simulink model "Firmodel"  (R2023b)
settings: Solver=VariableStepAuto  StartTime=0.0  StopTime=10.0  RelTol=1e-3
values from neighbouring files (symbols this model uses):
  ts = 1/fs    (= 4e-05)    [FIR.m]    (also in FIRfiltSam.m)
settings Model: Creator=91798  LastModifiedBy=91798
settings DataIOCC: ReturnWorkspaceOutputs=off

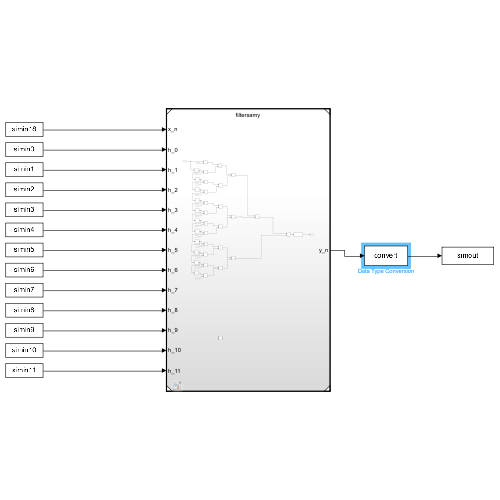
[thumbnail: Simulink's stored preview of the top-level diagram]
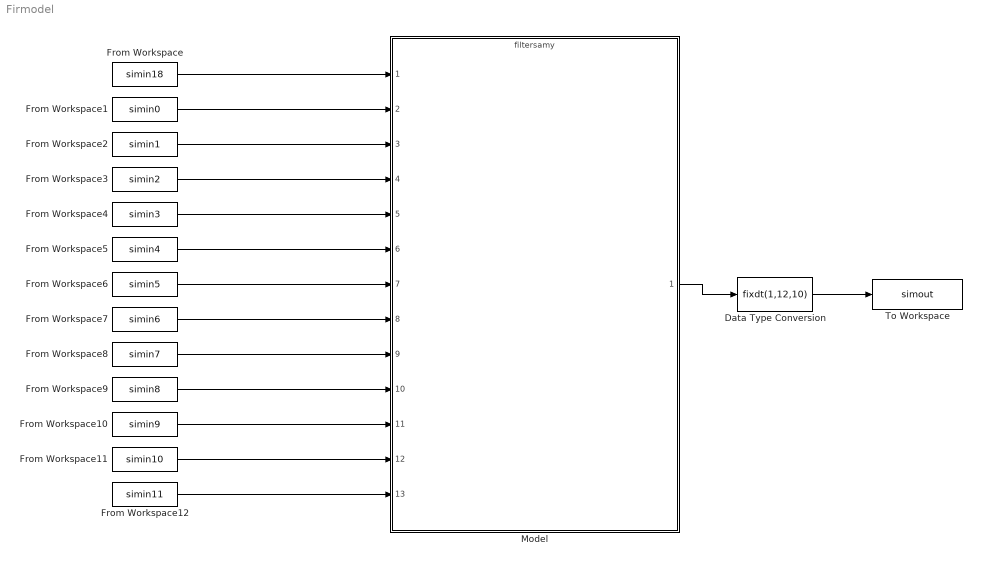
== system Firmodel ==
  Data Type Conversion : DataTypeConversion  OutDataTypeStr=fixdt(1,12,10)  SaturateOnIntegerOverflow=off  RndMeth=Floor
  From Workspace : FromWorkspace  VariableName=simin18  OutDataTypeStr=fixdt(1,8,6)  Interpolate=off  OutputAfterFinalValue=Setting to zero
  From Workspace1 : FromWorkspace  VariableName=simin0  OutDataTypeStr=fixdt(1,8,6)  Interpolate=off  OutputAfterFinalValue=Setting to zero
  From Workspace10 : FromWorkspace  VariableName=simin9  OutDataTypeStr=fixdt(1,8,6)  Interpolate=off  OutputAfterFinalValue=Setting to zero
  From Workspace11 : FromWorkspace  VariableName=simin10  OutDataTypeStr=fixdt(1,8,6)  SampleTime=ts  Interpolate=off  OutputAfterFinalValue=Setting to zero
  From Workspace12 : FromWorkspace  VariableName=simin11  OutDataTypeStr=fixdt(1,8,6)  Interpolate=off  OutputAfterFinalValue=Setting to zero
  From Workspace2 : FromWorkspace  VariableName=simin1  OutDataTypeStr=fixdt(1,8,6)  Interpolate=off  OutputAfterFinalValue=Setting to zero
  From Workspace3 : FromWorkspace  VariableName=simin2  OutDataTypeStr=fixdt(1,8,6)  Interpolate=off  OutputAfterFinalValue=Setting to zero
  From Workspace4 : FromWorkspace  VariableName=simin3  OutDataTypeStr=fixdt(1,8,6)  OutputAfterFinalValue=Setting to zero
  From Workspace5 : FromWorkspace  VariableName=simin4  OutDataTypeStr=fixdt(1,8,6)  Interpolate=off  OutputAfterFinalValue=Setting to zero
  From Workspace6 : FromWorkspace  VariableName=simin5  OutDataTypeStr=fixdt(1,8,6)  Interpolate=off  OutputAfterFinalValue=Setting to zero
  From Workspace7 : FromWorkspace  VariableName=simin6  OutDataTypeStr=fixdt(1,8,6)  Interpolate=off  OutputAfterFinalValue=Setting to zero
  From Workspace8 : FromWorkspace  VariableName=simin7  OutDataTypeStr=fixdt(1,8,6)  Interpolate=off  OutputAfterFinalValue=Setting to zero
  From Workspace9 : FromWorkspace  VariableName=simin8  OutDataTypeStr=fixdt(1,8,6)  Interpolate=off  OutputAfterFinalValue=Setting to zero
  Model : ModelReference  ModelNameDialog=filtersamy.slx  SimulationMode=Normal  ModelReferenceVersion=2.5
  To Workspace : ToWorkspace  VariableName=simout  SaveFormat=Timeseries  SampleTime=-1
  wires:
  From Workspace/1 -> Model/1
  From Workspace1/1 -> Model/2
  From Workspace2/1 -> Model/3
  From Workspace3/1 -> Model/4
  From Workspace4/1 -> Model/5
  From Workspace5/1 -> Model/6
  From Workspace6/1 -> Model/7
  From Workspace7/1 -> Model/8
  From Workspace8/1 -> Model/9
  From Workspace9/1 -> Model/10
  From Workspace10/1 -> Model/11
  From Workspace11/1 -> Model/12
  From Workspace12/1 -> Model/13
  Model/1 -> Data Type Conversion/1
  Data Type Conversion/1 -> To Workspace/1
